simulink model "Κυκλώματα_Ολοκληρωμένο"  (R2021a)
settings: Solver=ode23tb  StartTime=0.0  StopTime=0.10  MaxStep=1e-5  RelTol=1e-3
libraries: simulink x3, spsACVoltageSourceLib x1, spsCurrentMeasurementLib x1, eeGeneralControl x1, spsGroundLib x1, spsPowerLib x1, spsSeriesRLCBranchLib x1, spsVoltageMeasurementLib x1, spspowerguiLib x1
settings Model: Creator=epape  LastModifiedBy=epape

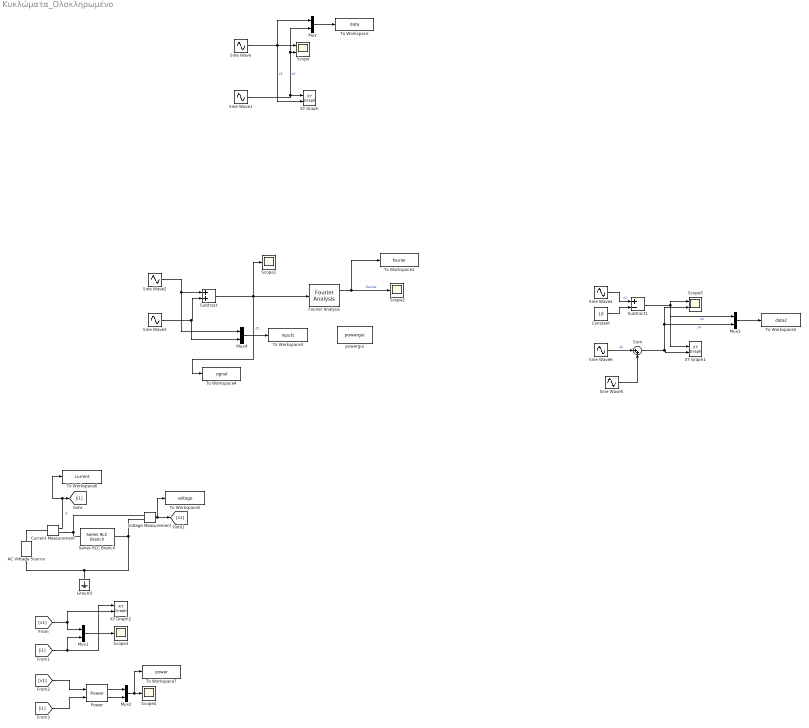
== system Κυκλώματα_Ολοκληρωμένο ==
  AC Voltage Source : spsACVoltageSourceLib/AC Voltage Source  Amplitude=230*sqrt(2)  Phase=90  Frequency=50  SampleTime=0  Measurements=Voltage  BusType=swing  Pref=10e3  Qref=0  Qmin=-inf  Qmax=+inf
  Constant : Constant  Value=10
  Current Measurement : spsCurrentMeasurementLib/Current Measurement  PhasorSimulation=off  OutputType=Complex  PSBequivalent=0
  Fourier Analysis : eeGeneralControl/Fourier Analysis  f=50  n=[1 2 3]  M0=0  Ph0=0  Ts=1e-5
      settings: SourceProductBaseCode=PS
  Ground : spsGroundLib/Ground  LConnTagsString=a
  Mux{,1..4} (5 alike) : Mux  Inputs=2
  Power : spsPowerLib/Power  Freq=50  Vinit=[1, 0]  Iinit=[1, 0]  Ts=0
      settings: SourceProductBaseCode=PS
  Scope : Scope  NumInputPorts=2
  Scope{1..4} (4 alike) : Scope
  Scope5 : Scope  NumInputPorts=2
  Series RLC Branch : spsSeriesRLCBranchLib/Series RLC Branch  LConnTagsString=__new0  RConnTagsString=__new0  BranchType=RL  Resistance=(23/2)*sqrt(3)  Inductance=(23/2)/(100*pi)  SetiL0=on  InitialCurrent=0  Capacitance=1e-6  Setx0=off  InitialVoltage=0  Measurements=None
  Sine Wave : Sin  Amplitude=100  Frequency=2*pi*50  SampleTime=0
  Sine Wave1 : Sin  Amplitude=100  Frequency=2*pi*50  Phase=pi/2  SampleTime=0
  Sine Wave2 : Sin  Amplitude=100  Frequency=2*pi*50  SampleTime=0
  Sine Wave3 : Sin  Amplitude=20  Frequency=2*pi*100  SampleTime=0
  Sine Wave4 : Sin  Amplitude=100  Frequency=2*pi*50  SampleTime=0
  Sine Wave5 : Sin  Amplitude=20  Frequency=2*pi*500  SampleTime=0
  Sine Wave6 : Sin  Amplitude=100  Frequency=2*pi*50  Phase=pi/2  SampleTime=0
  Subtract : Sum
  Subtract1 : Sum  Inputs=+-
  Sum : Sum  Inputs=|++
  To Workspace : ToWorkspace  VariableName=data  SaveFormat=Timeseries  SampleTime=1e-5
  To Workspace1 : ToWorkspace  VariableName=fourier  SaveFormat=Timeseries  SampleTime=1e-5
  To Workspace2 : ToWorkspace  VariableName=data2  SaveFormat=Timeseries  SampleTime=1e-5
  To Workspace3 : ToWorkspace  VariableName=inputs  SaveFormat=Timeseries  SampleTime=1e-5
  To Workspace4 : ToWorkspace  VariableName=signal  SaveFormat=Timeseries  SampleTime=1e-5
  To Workspace5 : ToWorkspace  VariableName=voltage  SaveFormat=Timeseries  SampleTime=1e-5
  To Workspace6 : ToWorkspace  VariableName=current  SaveFormat=Timeseries  SampleTime=1e-5
  To Workspace7 : ToWorkspace  VariableName=power  SaveFormat=Timeseries  SampleTime=1e-5
  Voltage Measurement : spsVoltageMeasurementLib/Voltage Measurement  PhasorSimulation=off  OutputType=Complex  PSBequivalent=0
  XY Graph : simulink/Sinks/XY Graph  xmin=-120  xmax=120  ymin=-120  ymax=120  st=-1
  XY Graph1 : simulink/Sinks/XY Graph  xmin=-150  xmax=150  ymin=-150  ymax=150  st=-1
  XY Graph2 : simulink/Sinks/XY Graph  xmin=-20  xmax=20  ymin=-350  ymax=350  st=-1
  powergui : spspowerguiLib/powergui  Priority=1  SimulationMode=Continuous  SampleTime=50e-6  frequency=60  Iterations=50  frequencyindice=50  Pbase=100e6  ErrMax=1e-4  UnitsV=kV  UnitsW=MW  buscounter=0  FunctionMessages=off  echomessages=off  EnableUseOfTLC=off  CurrentSourceSwitches=off  DisableSnubberDevices=off  DisableRonSwitches=off  DisableVfSwitches=off  DisplayEquations=off  AutomaticDiscreteSolvers=off  SolverType=Tustin/Backward Euler (TBE)  Interpol=off  ExternalGateDelay=off  methode=off  Ts=100  x0status=blocks  SPID=on  SwTol=0  HookPort=off  NonlinearTolerance=1e-4  nMaxIteration=100  ContinueOnMaxIteration=off  RestoreLinks=warning  ResistiveCurrentMeasurement=off  Frange=[0:2:500]  Ylog=off  Xlog=on  ShowGrid=off  save=off  variable=ZData  structure=0  ZoomFFT=off  StartTime=0.0  cycles=1  DisplayStyle=1  fundamental=60  FreqAxis=off  MaxFrequency=1000  frequencyindicesteady=1  RmsSteady=1  display=off
  wires:
  Sine Wave/1 -> Mux/1, XY Graph/2, Scope/1  "s1"
  Sine Wave1/1 -> Mux/2, Scope/2, XY Graph/1  "s2"
  Sine Wave2/1 -> Mux4/1, Subtract/1
  Sine Wave3/1 -> Mux4/2, Subtract/2
  Subtract/1 -> To Workspace4/1, Scope1/1, Fourier Analysis/1  "s5"
  Fourier Analysis/1 -> To Workspace1/1, Scope2/1  "fourier"
  Voltage Measurement/1 -> [v1], To Workspace5/1
  [v1] -> Mux1/1, XY Graph2/2
  [i1] -> XY Graph2/1, Mux1/2
  Mux1/1 -> Scope3/1
  [v1] -> Power/1
  [i1] -> Power/2
  Power/1 -> Mux2/1
  Power/2 -> Mux2/2
  Mux2/1 -> To Workspace7/1, Scope4/1
  Sine Wave4/1 -> Subtract1/1  "s1"
  Constant/1 -> Subtract1/2
  Sine Wave6/1 -> Sum/1  "s2"
  Sine Wave5/1 -> Sum/2
  Subtract1/1 -> Scope5/1, Mux3/1, XY Graph1/1  "s3"
  Sum/1 -> Mux3/2, Scope5/2, XY Graph1/2  "s4"
  Mux3/1 -> To Workspace2/1
  Mux4/1 -> To Workspace3/1
  Current Measurement/1 -> To Workspace6/1, [i1]  "i1"
  Mux/1 -> To Workspace/1
  connections:
  AC Voltage Source/LConn1 -- Voltage Measurement/LConn2 -- Series RLC Branch/RConn1 -- Ground/LConn1
  Voltage Measurement/LConn1 -- Current Measurement/RConn1 -- Series RLC Branch/LConn1
  AC Voltage Source/RConn1 -- Current Measurement/LConn1
